simulink model "InvertedPen"  (R2019b)
settings: Solver=VariableStepAuto  StartTime=0.0  StopTime=100.0  RelTol=1e-3
undefined symbols (not defined in the file): b, g, I, l, m, M
settings Model: Creator=ChiaYun  LastModifiedBy=15sin

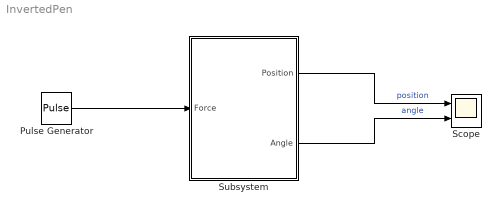
== system InvertedPen ==
  Pulse Generator : DiscretePulseGenerator  PulseType=Time based  Amplitude=1000  Period=10  PulseWidth=0.01
  Scope : Scope  NumInputPorts=2
  Subsystem : Subsystem
  wires:
  Pulse Generator/1 -> Subsystem/1(Force)
  Subsystem/1(Position) -> Scope/1  "position"
  Subsystem/2(Angle) -> Scope/2  "angle"

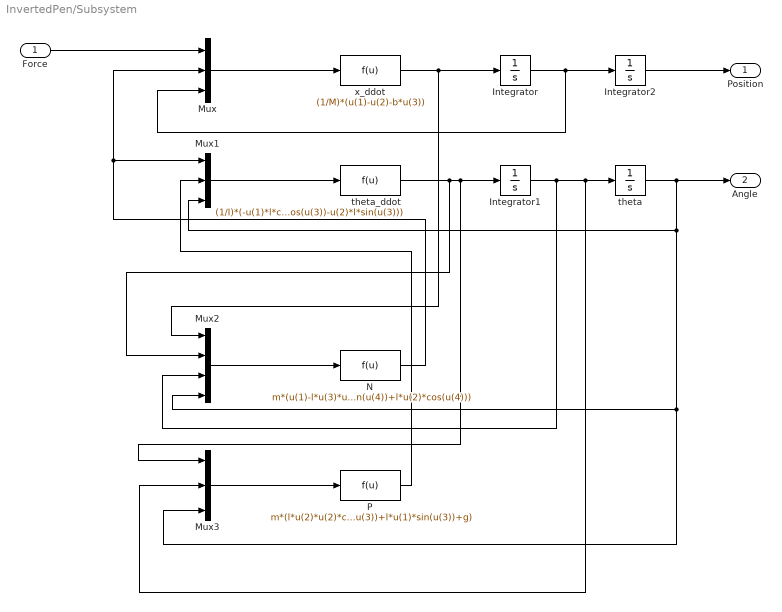
== system InvertedPen/Subsystem ==
  Force : Inport
  Integrator : Integrator
  Integrator1 : Integrator
  Integrator2 : Integrator
  Mux : Mux  Inputs=3
  Mux1 : Mux  Inputs=3
  Mux2 : Mux
  Mux3 : Mux  Inputs=3
  N : Fcn  Expr=m*(u(1)-l*u(3)*u(3)*sin(u(4))+l*u(2)*cos(u(4)))
  P : Fcn  Expr=m*(l*u(2)*u(2)*cos(u(3))+l*u(1)*sin(u(3))+g)
  theta : Integrator  InitialCondition=pi  ContinuousStateAttributes='theta'
  theta_ddot : Fcn  Expr=(1/I)*(-u(1)*l*cos(u(3))-u(2)*l*sin(u(3)))
  x_ddot : Fcn  Expr=(1/M)*(u(1)-u(2)-b*u(3))
  Position : Outport
  Angle : Outport  Port=2
  wires:
  P/1 -> Mux1/2
  Integrator/1 -> Mux/3, Integrator2/1
  N/1 -> Mux1/1, Mux/2
  theta_ddot/1 -> Mux2/2, Mux3/1, Integrator1/1
  Force/1 -> Mux/1
  theta/1 -> Angle/1, Mux3/3, Mux2/4, Mux1/3
  Mux/1 -> x_ddot/1
  Integrator1/1 -> Mux2/3, Mux3/2, theta/1
  Integrator2/1 -> Position/1
  Mux3/1 -> P/1
  Mux2/1 -> N/1
  x_ddot/1 -> Mux2/1, Integrator/1
  Mux1/1 -> theta_ddot/1
